simulink model "smotor2_1"  (Simulink 8.3)
settings: Solver=ode5  SolverMode=SingleTasking  StartTime=0.0  StopTime=5  FixedStep=0.001  RelTol=1e-3  AbsTol=1e-6
undefined symbols (not defined in the file or in its folder): bm, Jm, Kb, Kt, La, Ra
settings Model: Creator=ikko  LastModifiedBy=ikko
settings DataIOCC: LimitDataPoints=off  SignalLoggingName=logsOut
settings OptimizationCC: BooleanDataType=off  InitFltsAndDblsToZero=on
settings DebuggingCC: SaveWithParameterizedLinksMsg=none  CheckExecutionContextPreStartOutputMsg=on  CheckExecutionContextRuntimeOutputMsg=on  SignalResolutionControl=TryResolveAllWithWarning  SolverPrmCheckMsg=none  MultiTaskDSMMsg=warning  MultiTaskCondExecSysMsg=none  StateNameClashWarn=none  StrictBusMsg=None
settings HardwareCC: TargetUnknown=on
settings RTWCC: TemplateMakefile=grt_vc.tmf  IncludeERTFirstTime=on
settings GRTTargetCC: TargetFcnLib=ansi_tfl_tmw.mat

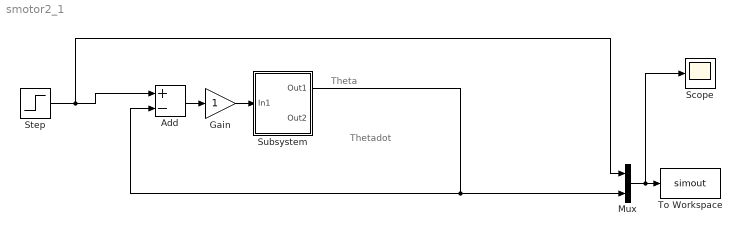
== system smotor2_1 ==
  note: Theta
  note: Thetadot
  Add : Sum  Inputs=+-
  Gain : Gain
  Mux : Mux  Inputs=2
  Scope : Scope
      settings: TickLabels=on
  Step : Step  SampleTime=0.001
  Subsystem : Subsystem
  To Workspace : ToWorkspace  VariableName=simout  SaveFormat=Structure  SampleTime=-1
  wires:
  Mux/1 -> To Workspace/1, Scope/1
  Add/1 -> Gain/1
  Step/1 -> Add/1, Mux/1
  Gain/1 -> Subsystem/1(In1)
  Subsystem/1(Out1) -> Mux/2, Add/2

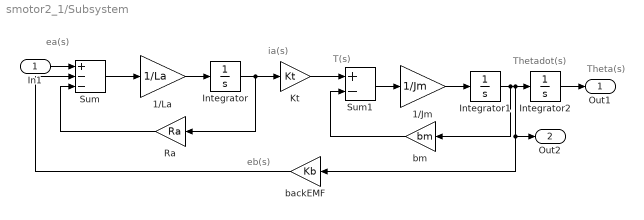
== system smotor2_1/Subsystem ==
  note: T(s)
  note: Theta(s)
  note: Thetadot(s)
  note: ea(s)
  note: eb(s)
  note: ia(s)
  In1 : Inport
  1/Jm : Gain  Gain=1/Jm  SaturateOnIntegerOverflow=on  OutDataTypeStr=Inherit: Same as input  ParamDataTypeStr=Inherit: Same as input
  1/La : Gain  Gain=1/La  SaturateOnIntegerOverflow=on  OutDataTypeStr=Inherit: Same as input  ParamDataTypeStr=Inherit: Same as input
  Integrator : Integrator
  Integrator1 : Integrator
  Integrator2 : Integrator
  Kt : Gain  Gain=Kt  SaturateOnIntegerOverflow=on  OutDataTypeStr=Inherit: Same as input  ParamDataTypeStr=Inherit: Same as input
  Ra : Gain  Gain=Ra  SaturateOnIntegerOverflow=on  OutDataTypeStr=Inherit: Same as input  ParamDataTypeStr=Inherit: Same as input
  Sum : Sum  Inputs=+--  SaturateOnIntegerOverflow=on  InputSameDT=on  OutDataTypeStr=Inherit: Same as first input
  Sum1 : Sum  Inputs=+-  SaturateOnIntegerOverflow=on  InputSameDT=on  OutDataTypeStr=Inherit: Same as first input
  backEMF : Gain  Gain=Kb  SaturateOnIntegerOverflow=on  OutDataTypeStr=Inherit: Same as input  ParamDataTypeStr=Inherit: Same as input
  bm : Gain  Gain=bm  SaturateOnIntegerOverflow=on  OutDataTypeStr=Inherit: Same as input  ParamDataTypeStr=Inherit: Same as input
  Out1 : Outport
  Out2 : Outport  Port=2
  wires:
  backEMF/1 -> Sum/2
  Kt/1 -> Sum1/1
  bm/1 -> Sum1/2
  Integrator1/1 -> backEMF/1, Out2/1, Integrator2/1, bm/1
  1/Jm/1 -> Integrator1/1
  Sum1/1 -> 1/Jm/1
  1/La/1 -> Integrator/1
  Sum/1 -> 1/La/1
  Ra/1 -> Sum/3
  Integrator/1 -> Ra/1, Kt/1
  In1/1 -> Sum/1
  Integrator2/1 -> Out1/1
